simulink model "DriveSystemControl"  (R2023b)
settings: Solver=FixedStepAuto  StartTime=0.0  StopTime=Inf  FixedStep=0.001  RelTol=1e-3
PostLoadFcn:
  | if any(exist('dsrtsu_mdlpostloadfcn', 'file') ~= 0), dsrtsu_mdlpostloadfcn('Execute', bdroot); end
InitFcn:
  | , if any(exist('rtifpga_mdlclblib', 'file') ~= 0), rtifpga_mdlclblib('Init', bdroot); end,
  | , if any(exist('dsmpb_private', 'file') ~= 0), dsmpb_private('dsmpb_mdlclblib', 'Init', bdroot); end,
libraries: dsmpblib x2
(part 5 of 11)

== system DriveSystemControl/Bus Configuration (1) - Out/Manipulation/Virya Controller CAN File 08082024/WIP/CANChannel/PDUs/TCU03/sigSupervisorFault ==
  sigSupervisorFault : Inport
  Feature Switch : Subsystem
  _sigSupervisorFault_ : BusSelector  OutputSignals=Feature Switch
  wires:
  sigSupervisorFault/1 -> _sigSupervisorFault_/1  "sigSupervisorFault"
  _sigSupervisorFault_/1 -> Feature Switch/1(Feature Switch)  "<Feature Switch>"

== system DriveSystemControl/Bus Configuration (1) - Out/Manipulation/Virya Controller CAN File 08082024/WIP/CANChannel/PDUs/TCU03/sigThrottlewiperHigh ==
  sigThrottlewiperHigh : Inport
  Feature Switch : Subsystem
  _sigThrottlewiperHigh_ : BusSelector  OutputSignals=Feature Switch
  wires:
  sigThrottlewiperHigh/1 -> _sigThrottlewiperHigh_/1  "sigThrottlewiperHigh"
  _sigThrottlewiperHigh_/1 -> Feature Switch/1(Feature Switch)  "<Feature Switch>"

== system DriveSystemControl/Bus Configuration (1) - Out/Manipulation/Virya Controller CAN File 08082024/WIP/CANChannel/PDUs/TCU03/sigThrottlewiperLow ==
  sigThrottlewiperLow : Inport
  Feature Switch : Subsystem
  _sigThrottlewiperLow_ : BusSelector  OutputSignals=Feature Switch
  wires:
  sigThrottlewiperLow/1 -> _sigThrottlewiperLow_/1  "sigThrottlewiperLow"
  _sigThrottlewiperLow_/1 -> Feature Switch/1(Feature Switch)  "<Feature Switch>"

== system DriveSystemControl/Bus Configuration (1) - Out/Manipulation/Virya Controller CAN File 08082024/WIP/CANChannel/PDUs/TCU03/sigVCLRunTimeError ==
  sigVCLRunTimeError : Inport
  Feature Switch : Subsystem
  _sigVCLRunTimeError_ : BusSelector  OutputSignals=Feature Switch
  wires:
  sigVCLRunTimeError/1 -> _sigVCLRunTimeError_/1  "sigVCLRunTimeError"
  _sigVCLRunTimeError_/1 -> Feature Switch/1(Feature Switch)  "<Feature Switch>"

== system DriveSystemControl/Bus Configuration (1) - Out/Manipulation/Virya Controller CAN File 08082024/WIP/CANChannel/PDUs/TCU04/sigMCU5_DriveMode ==
  sigMCU5_DriveMode : Inport
  Feature Switch : Subsystem
  _sigMCU5_DriveMode_ : BusSelector  OutputSignals=Feature Switch
  wires:
  sigMCU5_DriveMode/1 -> _sigMCU5_DriveMode_/1  "sigMCU5_DriveMode"
  _sigMCU5_DriveMode_/1 -> Feature Switch/1(Feature Switch)  "<Feature Switch>"

== system DriveSystemControl/Bus Configuration (1) - Out/Manipulation/Virya Controller CAN File 08082024/WIP/CANChannel/PDUs/TCU04/sigMCU5_Efficiency ==
  sigMCU5_Efficiency : Inport
  Feature Switch : Subsystem
  _sigMCU5_Efficiency_ : BusSelector  OutputSignals=Feature Switch
  wires:
  sigMCU5_Efficiency/1 -> _sigMCU5_Efficiency_/1  "sigMCU5_Efficiency"
  _sigMCU5_Efficiency_/1 -> Feature Switch/1(Feature Switch)  "<Feature Switch>"

== system DriveSystemControl/Bus Configuration (1) - Out/Manipulation/Virya Controller CAN File 08082024/WIP/CANChannel/PDUs/TCU04/sigMCU5_Hillhold ==
  sigMCU5_Hillhold : Inport
  Feature Switch : Subsystem
  _sigMCU5_Hillhold_ : BusSelector  OutputSignals=Feature Switch
  wires:
  sigMCU5_Hillhold/1 -> _sigMCU5_Hillhold_/1  "sigMCU5_Hillhold"
  _sigMCU5_Hillhold_/1 -> Feature Switch/1(Feature Switch)  "<Feature Switch>"

== system DriveSystemControl/Bus Configuration (1) - Out/Manipulation/Virya Controller CAN File 08082024/WIP/CANChannel/PDUs/TCU04/sigMCU5_RegenFlag ==
  sigMCU5_RegenFlag : Inport
  Feature Switch : Subsystem
  _sigMCU5_RegenFlag_ : BusSelector  OutputSignals=Feature Switch
  wires:
  sigMCU5_RegenFlag/1 -> _sigMCU5_RegenFlag_/1  "sigMCU5_RegenFlag"
  _sigMCU5_RegenFlag_/1 -> Feature Switch/1(Feature Switch)  "<Feature Switch>"

== system DriveSystemControl/Bus Configuration (1) - Out/Manipulation/Virya Controller CAN File 08082024/WIP/CANChannel/PDUs/TCU04/sigMCU5_Speed ==
  sigMCU5_Speed : Inport
  Feature Switch : Subsystem
  _sigMCU5_Speed_ : BusSelector  OutputSignals=Feature Switch
  wires:
  sigMCU5_Speed/1 -> _sigMCU5_Speed_/1  "sigMCU5_Speed"
  _sigMCU5_Speed_/1 -> Feature Switch/1(Feature Switch)  "<Feature Switch>"

== system DriveSystemControl/Bus Configuration (1) - Out/Manipulation/Virya Controller CAN File 08082024/WIP/CANChannel/PDUs/TCU05/sigMCU6_Odometer ==
  sigMCU6_Odometer : Inport
  Feature Switch : Subsystem
  _sigMCU6_Odometer_ : BusSelector  OutputSignals=Feature Switch
  wires:
  sigMCU6_Odometer/1 -> _sigMCU6_Odometer_/1  "sigMCU6_Odometer"
  _sigMCU6_Odometer_/1 -> Feature Switch/1(Feature Switch)  "<Feature Switch>"

== system DriveSystemControl/Bus Configuration (1) - Out/Simulated ECUs/Virya Controller CAN File 08082024/BMS/RX/PDUs/TCU04/sigMCU5_DriveMode ==
  sigMCU5_DriveMode : Inport
  ISignal Value : Subsystem
  _sigMCU5_DriveMode_ : BusSelector  OutputSignals=ISignal Value
  wires:
  sigMCU5_DriveMode/1 -> _sigMCU5_DriveMode_/1  "sigMCU5_DriveMode"
  _sigMCU5_DriveMode_/1 -> ISignal Value/1(ISignal Value)  "<ISignal Value>"

== system DriveSystemControl/Bus Configuration (1) - Out/Simulated ECUs/Virya Controller CAN File 08082024/BMS/RX/PDUs/TCU04/sigMCU5_Efficiency ==
  sigMCU5_Efficiency : Inport
  ISignal Value : Subsystem
  _sigMCU5_Efficiency_ : BusSelector  OutputSignals=ISignal Value
  wires:
  sigMCU5_Efficiency/1 -> _sigMCU5_Efficiency_/1  "sigMCU5_Efficiency"
  _sigMCU5_Efficiency_/1 -> ISignal Value/1(ISignal Value)  "<ISignal Value>"

== system DriveSystemControl/Bus Configuration (1) - Out/Simulated ECUs/Virya Controller CAN File 08082024/BMS/RX/PDUs/TCU04/sigMCU5_Hillhold ==
  sigMCU5_Hillhold : Inport
  ISignal Value : Subsystem
  _sigMCU5_Hillhold_ : BusSelector  OutputSignals=ISignal Value
  wires:
  sigMCU5_Hillhold/1 -> _sigMCU5_Hillhold_/1  "sigMCU5_Hillhold"
  _sigMCU5_Hillhold_/1 -> ISignal Value/1(ISignal Value)  "<ISignal Value>"

== system DriveSystemControl/Bus Configuration (1) - Out/Simulated ECUs/Virya Controller CAN File 08082024/BMS/RX/PDUs/TCU04/sigMCU5_RegenFlag ==
  sigMCU5_RegenFlag : Inport
  ISignal Value : Subsystem
  _sigMCU5_RegenFlag_ : BusSelector  OutputSignals=ISignal Value
  wires:
  sigMCU5_RegenFlag/1 -> _sigMCU5_RegenFlag_/1  "sigMCU5_RegenFlag"
  _sigMCU5_RegenFlag_/1 -> ISignal Value/1(ISignal Value)  "<ISignal Value>"

== system DriveSystemControl/Bus Configuration (1) - Out/Simulated ECUs/Virya Controller CAN File 08082024/BMS/RX/PDUs/TCU04/sigMCU5_Speed ==
  sigMCU5_Speed : Inport
  ISignal Value : Subsystem
  _sigMCU5_Speed_ : BusSelector  OutputSignals=ISignal Value
  wires:
  sigMCU5_Speed/1 -> _sigMCU5_Speed_/1  "sigMCU5_Speed"
  _sigMCU5_Speed_/1 -> ISignal Value/1(ISignal Value)  "<ISignal Value>"

== system DriveSystemControl/Bus Configuration (1) - Out/Simulated ECUs/Virya Controller CAN File 08082024/IPC/RX/PDUs/BMS01/sigBatteryMalfunctionLight ==
  sigBatteryMalfunctionLight : Inport
  ISignal Value : Subsystem
  _sigBatteryMalfunctionLight_ : BusSelector  OutputSignals=ISignal Value
  wires:
  sigBatteryMalfunctionLight/1 -> _sigBatteryMalfunctionLight_/1  "sigBatteryMalfunctionLight"
  _sigBatteryMalfunctionLight_/1 -> ISignal Value/1(ISignal Value)  "<ISignal Value>"

== system DriveSystemControl/Bus Configuration (1) - Out/Simulated ECUs/Virya Controller CAN File 08082024/IPC/RX/PDUs/BMS01/sigKeyOnIndicator ==
  sigKeyOnIndicator : Inport
  ISignal Value : Subsystem
  _sigKeyOnIndicator_ : BusSelector  OutputSignals=ISignal Value
  wires:
  sigKeyOnIndicator/1 -> _sigKeyOnIndicator_/1  "sigKeyOnIndicator"
  _sigKeyOnIndicator_/1 -> ISignal Value/1(ISignal Value)  "<ISignal Value>"

== system DriveSystemControl/Bus Configuration (1) - Out/Simulated ECUs/Virya Controller CAN File 08082024/IPC/RX/PDUs/BMS01/sigStateOfCharge ==
  sigStateOfCharge : Inport
  ISignal Value : Subsystem
  _sigStateOfCharge_ : BusSelector  OutputSignals=ISignal Value
  wires:
  sigStateOfCharge/1 -> _sigStateOfCharge_/1  "sigStateOfCharge"
  _sigStateOfCharge_/1 -> ISignal Value/1(ISignal Value)  "<ISignal Value>"

== system DriveSystemControl/Bus Configuration (1) - Out/Simulated ECUs/Virya Controller CAN File 08082024/IPC/RX/PDUs/TCU01/sigBrake ==
  sigBrake : Inport
  ISignal Value : Subsystem
  _sigBrake_ : BusSelector  OutputSignals=ISignal Value
  wires:
  sigBrake/1 -> _sigBrake_/1  "sigBrake"
  _sigBrake_/1 -> ISignal Value/1(ISignal Value)  "<ISignal Value>"

== system DriveSystemControl/Bus Configuration (1) - Out/Simulated ECUs/Virya Controller CAN File 08082024/IPC/RX/PDUs/TCU01/sigControllerTemperature ==
  sigControllerTemperature : Inport
  ISignal Value : Subsystem
  _sigControllerTemperature_ : BusSelector  OutputSignals=ISignal Value
  wires:
  sigControllerTemperature/1 -> _sigControllerTemperature_/1  "sigControllerTemperature"
  _sigControllerTemperature_/1 -> ISignal Value/1(ISignal Value)  "<ISignal Value>"

== system DriveSystemControl/Bus Configuration (1) - Out/Simulated ECUs/Virya Controller CAN File 08082024/IPC/RX/PDUs/TCU01/sigDriveMode ==
  sigDriveMode : Inport
  ISignal Value : Subsystem
  _sigDriveMode_ : BusSelector  OutputSignals=ISignal Value
  wires:
  sigDriveMode/1 -> _sigDriveMode_/1  "sigDriveMode"
  _sigDriveMode_/1 -> ISignal Value/1(ISignal Value)  "<ISignal Value>"

== system DriveSystemControl/Bus Configuration (1) - Out/Simulated ECUs/Virya Controller CAN File 08082024/IPC/RX/PDUs/TCU01/sigMotorTemperature ==
  sigMotorTemperature : Inport
  ISignal Value : Subsystem
  _sigMotorTemperature_ : BusSelector  OutputSignals=ISignal Value
  wires:
  sigMotorTemperature/1 -> _sigMotorTemperature_/1  "sigMotorTemperature"
  _sigMotorTemperature_/1 -> ISignal Value/1(ISignal Value)  "<ISignal Value>"

== system DriveSystemControl/Bus Configuration (1) - Out/Simulated ECUs/Virya Controller CAN File 08082024/IPC/RX/PDUs/TCU01/sigRMSCurrent ==
  sigRMSCurrent : Inport
  ISignal Value : Subsystem
  _sigRMSCurrent_ : BusSelector  OutputSignals=ISignal Value
  wires:
  sigRMSCurrent/1 -> _sigRMSCurrent_/1  "sigRMSCurrent"
  _sigRMSCurrent_/1 -> ISignal Value/1(ISignal Value)  "<ISignal Value>"

== system DriveSystemControl/Bus Configuration (1) - Out/Simulated ECUs/Virya Controller CAN File 08082024/IPC/RX/PDUs/TCU01/sigSpeed ==
  sigSpeed : Inport
  ISignal Value : Subsystem
  _sigSpeed_ : BusSelector  OutputSignals=ISignal Value
  wires:
  sigSpeed/1 -> _sigSpeed_/1  "sigSpeed"
  _sigSpeed_/1 -> ISignal Value/1(ISignal Value)  "<ISignal Value>"

== system DriveSystemControl/Bus Configuration (1) - Out/Simulated ECUs/Virya Controller CAN File 08082024/IPC/RX/PDUs/TCU01/sigThrottle ==
  sigThrottle : Inport
  ISignal Value : Subsystem
  _sigThrottle_ : BusSelector  OutputSignals=ISignal Value
  wires:
  sigThrottle/1 -> _sigThrottle_/1  "sigThrottle"
  _sigThrottle_/1 -> ISignal Value/1(ISignal Value)  "<ISignal Value>"

== system DriveSystemControl/Bus Configuration (1) - Out/Simulated ECUs/Virya Controller CAN File 08082024/IPC/RX/PDUs/TCU03/Controller_CompleteFaults ==
  Controller_CompleteFaults : Inport
  ISignal Value : Subsystem
  _Controller_CompleteFaults_ : BusSelector  OutputSignals=ISignal Value
  wires:
  Controller_CompleteFaults/1 -> _Controller_CompleteFaults_/1  "Controller_CompleteFaults"
  _Controller_CompleteFaults_/1 -> ISignal Value/1(ISignal Value)  "<ISignal Value>"

== system DriveSystemControl/Bus Configuration (1) - Out/Simulated ECUs/Virya Controller CAN File 08082024/IPC/RX/PDUs/TCU03/sig5VSupplyFailure ==
  sig5VSupplyFailure : Inport
  ISignal Value : Subsystem
  _sig5VSupplyFailure_ : BusSelector  OutputSignals=ISignal Value
  wires:
  sig5VSupplyFailure/1 -> _sig5VSupplyFailure_/1  "sig5VSupplyFailure"
  _sig5VSupplyFailure_/1 -> ISignal Value/1(ISignal Value)  "<ISignal Value>"

== system DriveSystemControl/Bus Configuration (1) - Out/Simulated ECUs/Virya Controller CAN File 08082024/IPC/RX/PDUs/TCU03/sigBPosOvervoltageCutback ==
  sigBPosOvervoltageCutback : Inport
  ISignal Value : Subsystem
  _sigBPosOvervoltageCutback_ : BusSelector  OutputSignals=ISignal Value
  wires:
  sigBPosOvervoltageCutback/1 -> _sigBPosOvervoltageCutback_/1  "sigBPosOvervoltageCutback"
  _sigBPosOvervoltageCutback_/1 -> ISignal Value/1(ISignal Value)  "<ISignal Value>"

== system DriveSystemControl/Bus Configuration (1) - Out/Simulated ECUs/Virya Controller CAN File 08082024/IPC/RX/PDUs/TCU03/sigBPosUndervoltageCutback ==
  sigBPosUndervoltageCutback : Inport
  ISignal Value : Subsystem
  _sigBPosUndervoltageCutback_ : BusSelector  OutputSignals=ISignal Value
  wires:
  sigBPosUndervoltageCutback/1 -> _sigBPosUndervoltageCutback_/1  "sigBPosUndervoltageCutback"
  _sigBPosUndervoltageCutback_/1 -> ISignal Value/1(ISignal Value)  "<ISignal Value>"

== system DriveSystemControl/Bus Configuration (1) - Out/Simulated ECUs/Virya Controller CAN File 08082024/IPC/RX/PDUs/TCU03/sigBadCalibration ==
  sigBadCalibration : Inport
  ISignal Value : Subsystem
  _sigBadCalibration_ : BusSelector  OutputSignals=ISignal Value
  wires:
  sigBadCalibration/1 -> _sigBadCalibration_/1  "sigBadCalibration"
  _sigBadCalibration_/1 -> ISignal Value/1(ISignal Value)  "<ISignal Value>"

== system DriveSystemControl/Bus Configuration (1) - Out/Simulated ECUs/Virya Controller CAN File 08082024/IPC/RX/PDUs/TCU03/sigBrakeWiperHigh ==
  sigBrakeWiperHigh : Inport
  ISignal Value : Subsystem
  _sigBrakeWiperHigh_ : BusSelector  OutputSignals=ISignal Value
  wires:
  sigBrakeWiperHigh/1 -> _sigBrakeWiperHigh_/1  "sigBrakeWiperHigh"
  _sigBrakeWiperHigh_/1 -> ISignal Value/1(ISignal Value)  "<ISignal Value>"

== system DriveSystemControl/Bus Configuration (1) - Out/Simulated ECUs/Virya Controller CAN File 08082024/IPC/RX/PDUs/TCU03/sigBrakeWiperLow ==
  sigBrakeWiperLow : Inport
  ISignal Value : Subsystem
  _sigBrakeWiperLow_ : BusSelector  OutputSignals=ISignal Value
  wires:
  sigBrakeWiperLow/1 -> _sigBrakeWiperLow_/1  "sigBrakeWiperLow"
  _sigBrakeWiperLow_/1 -> ISignal Value/1(ISignal Value)  "<ISignal Value>"

== system DriveSystemControl/Bus Configuration (1) - Out/Simulated ECUs/Virya Controller CAN File 08082024/IPC/RX/PDUs/TCU03/sigCoil2DriverOpenShort ==
  sigCoil2DriverOpenShort : Inport
  ISignal Value : Subsystem
  _sigCoil2DriverOpenShort_ : BusSelector  OutputSignals=ISignal Value
  wires:
  sigCoil2DriverOpenShort/1 -> _sigCoil2DriverOpenShort_/1  "sigCoil2DriverOpenShort"
  _sigCoil2DriverOpenShort_/1 -> ISignal Value/1(ISignal Value)  "<ISignal Value>"

== system DriveSystemControl/Bus Configuration (1) - Out/Simulated ECUs/Virya Controller CAN File 08082024/IPC/RX/PDUs/TCU03/sigCoil3DriverOpenShort ==
  sigCoil3DriverOpenShort : Inport
  ISignal Value : Subsystem
  _sigCoil3DriverOpenShort_ : BusSelector  OutputSignals=ISignal Value
  wires:
  sigCoil3DriverOpenShort/1 -> _sigCoil3DriverOpenShort_/1  "sigCoil3DriverOpenShort"
  _sigCoil3DriverOpenShort_/1 -> ISignal Value/1(ISignal Value)  "<ISignal Value>"

== system DriveSystemControl/Bus Configuration (1) - Out/Simulated ECUs/Virya Controller CAN File 08082024/IPC/RX/PDUs/TCU03/sigCoil4DriverOpenShort ==
  sigCoil4DriverOpenShort : Inport
  ISignal Value : Subsystem
  _sigCoil4DriverOpenShort_ : BusSelector  OutputSignals=ISignal Value
  wires:
  sigCoil4DriverOpenShort/1 -> _sigCoil4DriverOpenShort_/1  "sigCoil4DriverOpenShort"
  _sigCoil4DriverOpenShort_/1 -> ISignal Value/1(ISignal Value)  "<ISignal Value>"

== system DriveSystemControl/Bus Configuration (1) - Out/Simulated ECUs/Virya Controller CAN File 08082024/IPC/RX/PDUs/TCU03/sigControllerCommonFault ==
  sigControllerCommonFault : Inport
  ISignal Value : Subsystem
  _sigControllerCommonFault_ : BusSelector  OutputSignals=ISignal Value
  wires:
  sigControllerCommonFault/1 -> _sigControllerCommonFault_/1  "sigControllerCommonFault"
  _sigControllerCommonFault_/1 -> ISignal Value/1(ISignal Value)  "<ISignal Value>"

== system DriveSystemControl/Bus Configuration (1) - Out/Simulated ECUs/Virya Controller CAN File 08082024/IPC/RX/PDUs/TCU03/sigControllerOverCurrent ==
  sigControllerOverCurrent : Inport
  ISignal Value : Subsystem
  _sigControllerOverCurrent_ : BusSelector  OutputSignals=ISignal Value
  wires:
  sigControllerOverCurrent/1 -> _sigControllerOverCurrent_/1  "sigControllerOverCurrent"
  _sigControllerOverCurrent_/1 -> ISignal Value/1(ISignal Value)  "<ISignal Value>"

== system DriveSystemControl/Bus Configuration (1) - Out/Simulated ECUs/Virya Controller CAN File 08082024/IPC/RX/PDUs/TCU03/sigControllerOvertempCutback ==
  sigControllerOvertempCutback : Inport
  ISignal Value : Subsystem
  _sigControllerOvertempCutback_ : BusSelector  OutputSignals=ISignal Value
  wires:
  sigControllerOvertempCutback/1 -> _sigControllerOvertempCutback_/1  "sigControllerOvertempCutback"
  _sigControllerOvertempCutback_/1 -> ISignal Value/1(ISignal Value)  "<ISignal Value>"

== system DriveSystemControl/Bus Configuration (1) - Out/Simulated ECUs/Virya Controller CAN File 08082024/IPC/RX/PDUs/TCU03/sigControllerSevereOvertemp ==
  sigControllerSevereOvertemp : Inport
  ISignal Value : Subsystem
  _sigControllerSevereOvertemp_ : BusSelector  OutputSignals=ISignal Value
  wires:
  sigControllerSevereOvertemp/1 -> _sigControllerSevereOvertemp_/1  "sigControllerSevereOvertemp"
  _sigControllerSevereOvertemp_/1 -> ISignal Value/1(ISignal Value)  "<ISignal Value>"

== system DriveSystemControl/Bus Configuration (1) - Out/Simulated ECUs/Virya Controller CAN File 08082024/IPC/RX/PDUs/TCU03/sigControllerSevereUndertemp ==
  sigControllerSevereUndertemp : Inport
  ISignal Value : Subsystem
  _sigControllerSevereUndertemp_ : BusSelector  OutputSignals=ISignal Value
  wires:
  sigControllerSevereUndertemp/1 -> _sigControllerSevereUndertemp_/1  "sigControllerSevereUndertemp"
  _sigControllerSevereUndertemp_/1 -> ISignal Value/1(ISignal Value)  "<ISignal Value>"

== system DriveSystemControl/Bus Configuration (1) - Out/Simulated ECUs/Virya Controller CAN File 08082024/IPC/RX/PDUs/TCU03/sigCurrentSensorFault ==
  sigCurrentSensorFault : Inport
  ISignal Value : Subsystem
  _sigCurrentSensorFault_ : BusSelector  OutputSignals=ISignal Value
  wires:
  sigCurrentSensorFault/1 -> _sigCurrentSensorFault_/1  "sigCurrentSensorFault"
  _sigCurrentSensorFault_/1 -> ISignal Value/1(ISignal Value)  "<ISignal Value>"

== system DriveSystemControl/Bus Configuration (1) - Out/Simulated ECUs/Virya Controller CAN File 08082024/IPC/RX/PDUs/TCU03/sigEEPROMFailure ==
  sigEEPROMFailure : Inport
  ISignal Value : Subsystem
  _sigEEPROMFailure_ : BusSelector  OutputSignals=ISignal Value
  wires:
  sigEEPROMFailure/1 -> _sigEEPROMFailure_/1  "sigEEPROMFailure"
  _sigEEPROMFailure_/1 -> ISignal Value/1(ISignal Value)  "<ISignal Value>"

== system DriveSystemControl/Bus Configuration (1) - Out/Simulated ECUs/Virya Controller CAN File 08082024/IPC/RX/PDUs/TCU03/sigHighPedalDisable ==
  sigHighPedalDisable : Inport
  ISignal Value : Subsystem
  _sigHighPedalDisable_ : BusSelector  OutputSignals=ISignal Value
  wires:
  sigHighPedalDisable/1 -> _sigHighPedalDisable_/1  "sigHighPedalDisable"
  _sigHighPedalDisable_/1 -> ISignal Value/1(ISignal Value)  "<ISignal Value>"

== system DriveSystemControl/Bus Configuration (1) - Out/Simulated ECUs/Virya Controller CAN File 08082024/IPC/RX/PDUs/TCU03/sigInsulationResistanceLow ==
  sigInsulationResistanceLow : Inport
  ISignal Value : Subsystem
  _sigInsulationResistanceLow_ : BusSelector  OutputSignals=ISignal Value
  wires:
  sigInsulationResistanceLow/1 -> _sigInsulationResistanceLow_/1  "sigInsulationResistanceLow"
  _sigInsulationResistanceLow_/1 -> ISignal Value/1(ISignal Value)  "<ISignal Value>"

== system DriveSystemControl/Bus Configuration (1) - Out/Simulated ECUs/Virya Controller CAN File 08082024/IPC/RX/PDUs/TCU03/sigMainContactorWelded ==
  sigMainContactorWelded : Inport
  ISignal Value : Subsystem
  _sigMainContactorWelded_ : BusSelector  OutputSignals=ISignal Value
  wires:
  sigMainContactorWelded/1 -> _sigMainContactorWelded_/1  "sigMainContactorWelded"
  _sigMainContactorWelded_/1 -> ISignal Value/1(ISignal Value)  "<ISignal Value>"

== system DriveSystemControl/Bus Configuration (1) - Out/Simulated ECUs/Virya Controller CAN File 08082024/IPC/RX/PDUs/TCU03/sigMainContactordidnotClose ==
  sigMainContactordidnotClose : Inport
  ISignal Value : Subsystem
  _sigMainContactordidnotClose_ : BusSelector  OutputSignals=ISignal Value
  wires:
  sigMainContactordidnotClose/1 -> _sigMainContactordidnotClose_/1  "sigMainContactordidnotClose"
  _sigMainContactordidnotClose_/1 -> ISignal Value/1(ISignal Value)  "<ISignal Value>"

== system DriveSystemControl/Bus Configuration (1) - Out/Simulated ECUs/Virya Controller CAN File 08082024/IPC/RX/PDUs/TCU03/sigMainOpenShort ==
  sigMainOpenShort : Inport
  ISignal Value : Subsystem
  _sigMainOpenShort_ : BusSelector  OutputSignals=ISignal Value
  wires:
  sigMainOpenShort/1 -> _sigMainOpenShort_/1  "sigMainOpenShort"
  _sigMainOpenShort_/1 -> ISignal Value/1(ISignal Value)  "<ISignal Value>"

== system DriveSystemControl/Bus Configuration (1) - Out/Simulated ECUs/Virya Controller CAN File 08082024/IPC/RX/PDUs/TCU03/sigMotorCharacterization ==
  sigMotorCharacterization : Inport
  ISignal Value : Subsystem
  _sigMotorCharacterization_ : BusSelector  OutputSignals=ISignal Value
  wires:
  sigMotorCharacterization/1 -> _sigMotorCharacterization_/1  "sigMotorCharacterization"
  _sigMotorCharacterization_/1 -> ISignal Value/1(ISignal Value)  "<ISignal Value>"

== system DriveSystemControl/Bus Configuration (1) - Out/Simulated ECUs/Virya Controller CAN File 08082024/IPC/RX/PDUs/TCU03/sigMotorPhaseOpen ==
  sigMotorPhaseOpen : Inport
  ISignal Value : Subsystem
  _sigMotorPhaseOpen_ : BusSelector  OutputSignals=ISignal Value
  wires:
  sigMotorPhaseOpen/1 -> _sigMotorPhaseOpen_/1  "sigMotorPhaseOpen"
  _sigMotorPhaseOpen_/1 -> ISignal Value/1(ISignal Value)  "<ISignal Value>"

== system DriveSystemControl/Bus Configuration (1) - Out/Simulated ECUs/Virya Controller CAN File 08082024/IPC/RX/PDUs/TCU03/sigMotorTempHotCutback ==
  sigMotorTempHotCutback : Inport
  ISignal Value : Subsystem
  _sigMotorTempHotCutback_ : BusSelector  OutputSignals=ISignal Value
  wires:
  sigMotorTempHotCutback/1 -> _sigMotorTempHotCutback_/1  "sigMotorTempHotCutback"
  _sigMotorTempHotCutback_/1 -> ISignal Value/1(ISignal Value)  "<ISignal Value>"

== system DriveSystemControl/Bus Configuration (1) - Out/Simulated ECUs/Virya Controller CAN File 08082024/IPC/RX/PDUs/TCU03/sigMotorTempSensorFault ==
  sigMotorTempSensorFault : Inport
  ISignal Value : Subsystem
  _sigMotorTempSensorFault_ : BusSelector  OutputSignals=ISignal Value
  wires:
  sigMotorTempSensorFault/1 -> _sigMotorTempSensorFault_/1  "sigMotorTempSensorFault"
  _sigMotorTempSensorFault_/1 -> ISignal Value/1(ISignal Value)  "<ISignal Value>"

== system DriveSystemControl/Bus Configuration (1) - Out/Simulated ECUs/Virya Controller CAN File 08082024/IPC/RX/PDUs/TCU03/sigOEM_BatterySTOPSignal ==
  sigOEM_BatterySTOPSignal : Inport
  ISignal Value : Subsystem
  _sigOEM_BatterySTOPSignal_ : BusSelector  OutputSignals=ISignal Value
  wires:
  sigOEM_BatterySTOPSignal/1 -> _sigOEM_BatterySTOPSignal_/1  "sigOEM_BatterySTOPSignal"
  _sigOEM_BatterySTOPSignal_/1 -> ISignal Value/1(ISignal Value)  "<ISignal Value>"

== system DriveSystemControl/Bus Configuration (1) - Out/Simulated ECUs/Virya Controller CAN File 08082024/IPC/RX/PDUs/TCU03/sigOEM_NoBatteryCAN ==
  sigOEM_NoBatteryCAN : Inport
  ISignal Value : Subsystem
  _sigOEM_NoBatteryCAN_ : BusSelector  OutputSignals=ISignal Value
  wires:
  sigOEM_NoBatteryCAN/1 -> _sigOEM_NoBatteryCAN_/1  "sigOEM_NoBatteryCAN"
  _sigOEM_NoBatteryCAN_/1 -> ISignal Value/1(ISignal Value)  "<ISignal Value>"

== system DriveSystemControl/Bus Configuration (1) - Out/Simulated ECUs/Virya Controller CAN File 08082024/IPC/RX/PDUs/TCU03/sigOSGeneral ==
  sigOSGeneral : Inport
  ISignal Value : Subsystem
  _sigOSGeneral_ : BusSelector  OutputSignals=ISignal Value
  wires:
  sigOSGeneral/1 -> _sigOSGeneral_/1  "sigOSGeneral"
  _sigOSGeneral_/1 -> ISignal Value/1(ISignal Value)  "<ISignal Value>"

== system DriveSystemControl/Bus Configuration (1) - Out/Simulated ECUs/Virya Controller CAN File 08082024/IPC/RX/PDUs/TCU03/sigPMACCommissioningNeeded ==
  sigPMACCommissioningNeeded : Inport
  ISignal Value : Subsystem
  _sigPMACCommissioningNeeded_ : BusSelector  OutputSignals=ISignal Value
  wires:
  sigPMACCommissioningNeeded/1 -> _sigPMACCommissioningNeeded_/1  "sigPMACCommissioningNeeded"
  _sigPMACCommissioningNeeded_/1 -> ISignal Value/1(ISignal Value)  "<ISignal Value>"

== system DriveSystemControl/Bus Configuration (1) - Out/Simulated ECUs/Virya Controller CAN File 08082024/IPC/RX/PDUs/TCU03/sigParameterChangeFault ==
  sigParameterChangeFault : Inport
  ISignal Value : Subsystem
  _sigParameterChangeFault_ : BusSelector  OutputSignals=ISignal Value
  wires:
  sigParameterChangeFault/1 -> _sigParameterChangeFault_/1  "sigParameterChangeFault"
  _sigParameterChangeFault_/1 -> ISignal Value/1(ISignal Value)  "<ISignal Value>"

== system DriveSystemControl/Bus Configuration (1) - Out/Simulated ECUs/Virya Controller CAN File 08082024/IPC/RX/PDUs/TCU03/sigPhasePWMMismatch ==
  sigPhasePWMMismatch : Inport
  ISignal Value : Subsystem
  _sigPhasePWMMismatch_ : BusSelector  OutputSignals=ISignal Value
  wires:
  sigPhasePWMMismatch/1 -> _sigPhasePWMMismatch_/1  "sigPhasePWMMismatch"
  _sigPhasePWMMismatch_/1 -> ISignal Value/1(ISignal Value)  "<ISignal Value>"

== system DriveSystemControl/Bus Configuration (1) - Out/Simulated ECUs/Virya Controller CAN File 08082024/IPC/RX/PDUs/TCU03/sigPrechargeFailed ==
  sigPrechargeFailed : Inport
  ISignal Value : Subsystem
  _sigPrechargeFailed_ : BusSelector  OutputSignals=ISignal Value
  wires:
  sigPrechargeFailed/1 -> _sigPrechargeFailed_/1  "sigPrechargeFailed"
  _sigPrechargeFailed_/1 -> ISignal Value/1(ISignal Value)  "<ISignal Value>"

== system DriveSystemControl/Bus Configuration (1) - Out/Simulated ECUs/Virya Controller CAN File 08082024/IPC/RX/PDUs/TCU03/sigSevereBPosOvervoltage ==
  sigSevereBPosOvervoltage : Inport
  ISignal Value : Subsystem
  _sigSevereBPosOvervoltage_ : BusSelector  OutputSignals=ISignal Value
  wires:
  sigSevereBPosOvervoltage/1 -> _sigSevereBPosOvervoltage_/1  "sigSevereBPosOvervoltage"
  _sigSevereBPosOvervoltage_/1 -> ISignal Value/1(ISignal Value)  "<ISignal Value>"

== system DriveSystemControl/Bus Configuration (1) - Out/Simulated ECUs/Virya Controller CAN File 08082024/IPC/RX/PDUs/TCU03/sigSevereBPosUndervoltage ==
  sigSevereBPosUndervoltage : Inport
  ISignal Value : Subsystem
  _sigSevereBPosUndervoltage_ : BusSelector  OutputSignals=ISignal Value
  wires:
  sigSevereBPosUndervoltage/1 -> _sigSevereBPosUndervoltage_/1  "sigSevereBPosUndervoltage"
  _sigSevereBPosUndervoltage_/1 -> ISignal Value/1(ISignal Value)  "<ISignal Value>"

== system DriveSystemControl/Bus Configuration (1) - Out/Simulated ECUs/Virya Controller CAN File 08082024/IPC/RX/PDUs/TCU03/sigSevereKSIOvervoltage ==
  sigSevereKSIOvervoltage : Inport
  ISignal Value : Subsystem
  _sigSevereKSIOvervoltage_ : BusSelector  OutputSignals=ISignal Value
  wires:
  sigSevereKSIOvervoltage/1 -> _sigSevereKSIOvervoltage_/1  "sigSevereKSIOvervoltage"
  _sigSevereKSIOvervoltage_/1 -> ISignal Value/1(ISignal Value)  "<ISignal Value>"

== system DriveSystemControl/Bus Configuration (1) - Out/Simulated ECUs/Virya Controller CAN File 08082024/IPC/RX/PDUs/TCU03/sigSevereKSIUndervoltage ==
  sigSevereKSIUndervoltage : Inport
  ISignal Value : Subsystem
  _sigSevereKSIUndervoltage_ : BusSelector  OutputSignals=ISignal Value
  wires:
  sigSevereKSIUndervoltage/1 -> _sigSevereKSIUndervoltage_/1  "sigSevereKSIUndervoltage"
  _sigSevereKSIUndervoltage_/1 -> ISignal Value/1(ISignal Value)  "<ISignal Value>"

== system DriveSystemControl/Bus Configuration (1) - Out/Simulated ECUs/Virya Controller CAN File 08082024/IPC/RX/PDUs/TCU03/sigSinCosMisalignment ==
  sigSinCosMisalignment : Inport
  ISignal Value : Subsystem
  _sigSinCosMisalignment_ : BusSelector  OutputSignals=ISignal Value
  wires:
  sigSinCosMisalignment/1 -> _sigSinCosMisalignment_/1  "sigSinCosMisalignment"
  _sigSinCosMisalignment_/1 -> ISignal Value/1(ISignal Value)  "<ISignal Value>"

== system DriveSystemControl/Bus Configuration (1) - Out/Simulated ECUs/Virya Controller CAN File 08082024/IPC/RX/PDUs/TCU03/sigSinCosSensorFault ==
  sigSinCosSensorFault : Inport
  ISignal Value : Subsystem
  _sigSinCosSensorFault_ : BusSelector  OutputSignals=ISignal Value
  wires:
  sigSinCosSensorFault/1 -> _sigSinCosSensorFault_/1  "sigSinCosSensorFault"
  _sigSinCosSensorFault_/1 -> ISignal Value/1(ISignal Value)  "<ISignal Value>"

== system DriveSystemControl/Bus Configuration (1) - Out/Simulated ECUs/Virya Controller CAN File 08082024/IPC/RX/PDUs/TCU03/sigStallDetected ==
  sigStallDetected : Inport
  ISignal Value : Subsystem
  _sigStallDetected_ : BusSelector  OutputSignals=ISignal Value
  wires:
  sigStallDetected/1 -> _sigStallDetected_/1  "sigStallDetected"
  _sigStallDetected_/1 -> ISignal Value/1(ISignal Value)  "<ISignal Value>"

== system DriveSystemControl/Bus Configuration (1) - Out/Simulated ECUs/Virya Controller CAN File 08082024/IPC/RX/PDUs/TCU03/sigSupervisorFault ==
  sigSupervisorFault : Inport
  ISignal Value : Subsystem
  _sigSupervisorFault_ : BusSelector  OutputSignals=ISignal Value
  wires:
  sigSupervisorFault/1 -> _sigSupervisorFault_/1  "sigSupervisorFault"
  _sigSupervisorFault_/1 -> ISignal Value/1(ISignal Value)  "<ISignal Value>"

== system DriveSystemControl/Bus Configuration (1) - Out/Simulated ECUs/Virya Controller CAN File 08082024/IPC/RX/PDUs/TCU03/sigThrottlewiperHigh ==
  sigThrottlewiperHigh : Inport
  ISignal Value : Subsystem
  _sigThrottlewiperHigh_ : BusSelector  OutputSignals=ISignal Value
  wires:
  sigThrottlewiperHigh/1 -> _sigThrottlewiperHigh_/1  "sigThrottlewiperHigh"
  _sigThrottlewiperHigh_/1 -> ISignal Value/1(ISignal Value)  "<ISignal Value>"

== system DriveSystemControl/Bus Configuration (1) - Out/Simulated ECUs/Virya Controller CAN File 08082024/IPC/RX/PDUs/TCU03/sigThrottlewiperLow ==
  sigThrottlewiperLow : Inport
  ISignal Value : Subsystem
  _sigThrottlewiperLow_ : BusSelector  OutputSignals=ISignal Value
  wires:
  sigThrottlewiperLow/1 -> _sigThrottlewiperLow_/1  "sigThrottlewiperLow"
  _sigThrottlewiperLow_/1 -> ISignal Value/1(ISignal Value)  "<ISignal Value>"

== system DriveSystemControl/Bus Configuration (1) - Out/Simulated ECUs/Virya Controller CAN File 08082024/IPC/RX/PDUs/TCU03/sigVCLRunTimeError ==
  sigVCLRunTimeError : Inport
  ISignal Value : Subsystem
  _sigVCLRunTimeError_ : BusSelector  OutputSignals=ISignal Value
  wires:
  sigVCLRunTimeError/1 -> _sigVCLRunTimeError_/1  "sigVCLRunTimeError"
  _sigVCLRunTimeError_/1 -> ISignal Value/1(ISignal Value)  "<ISignal Value>"

== system DriveSystemControl/Bus Configuration (1) - Out/Simulated ECUs/Virya Controller CAN File 08082024/IPC/RX/PDUs/TCU04/sigMCU5_DriveMode ==
  sigMCU5_DriveMode : Inport
  ISignal Value : Subsystem
  _sigMCU5_DriveMode_ : BusSelector  OutputSignals=ISignal Value
  wires:
  sigMCU5_DriveMode/1 -> _sigMCU5_DriveMode_/1  "sigMCU5_DriveMode"
  _sigMCU5_DriveMode_/1 -> ISignal Value/1(ISignal Value)  "<ISignal Value>"

== system DriveSystemControl/Bus Configuration (1) - Out/Simulated ECUs/Virya Controller CAN File 08082024/IPC/RX/PDUs/TCU04/sigMCU5_Efficiency ==
  sigMCU5_Efficiency : Inport
  ISignal Value : Subsystem
  _sigMCU5_Efficiency_ : BusSelector  OutputSignals=ISignal Value
  wires:
  sigMCU5_Efficiency/1 -> _sigMCU5_Efficiency_/1  "sigMCU5_Efficiency"
  _sigMCU5_Efficiency_/1 -> ISignal Value/1(ISignal Value)  "<ISignal Value>"

== system DriveSystemControl/Bus Configuration (1) - Out/Simulated ECUs/Virya Controller CAN File 08082024/IPC/RX/PDUs/TCU04/sigMCU5_Hillhold ==
  sigMCU5_Hillhold : Inport
  ISignal Value : Subsystem
  _sigMCU5_Hillhold_ : BusSelector  OutputSignals=ISignal Value
  wires:
  sigMCU5_Hillhold/1 -> _sigMCU5_Hillhold_/1  "sigMCU5_Hillhold"
  _sigMCU5_Hillhold_/1 -> ISignal Value/1(ISignal Value)  "<ISignal Value>"

== system DriveSystemControl/Bus Configuration (1) - Out/Simulated ECUs/Virya Controller CAN File 08082024/IPC/RX/PDUs/TCU04/sigMCU5_RegenFlag ==
  sigMCU5_RegenFlag : Inport
  ISignal Value : Subsystem
  _sigMCU5_RegenFlag_ : BusSelector  OutputSignals=ISignal Value
  wires:
  sigMCU5_RegenFlag/1 -> _sigMCU5_RegenFlag_/1  "sigMCU5_RegenFlag"
  _sigMCU5_RegenFlag_/1 -> ISignal Value/1(ISignal Value)  "<ISignal Value>"

== system DriveSystemControl/Bus Configuration (1) - Out/Simulated ECUs/Virya Controller CAN File 08082024/IPC/RX/PDUs/TCU04/sigMCU5_Speed ==
  sigMCU5_Speed : Inport
  ISignal Value : Subsystem
  _sigMCU5_Speed_ : BusSelector  OutputSignals=ISignal Value
  wires:
  sigMCU5_Speed/1 -> _sigMCU5_Speed_/1  "sigMCU5_Speed"
  _sigMCU5_Speed_/1 -> ISignal Value/1(ISignal Value)  "<ISignal Value>"

== system DriveSystemControl/Bus Configuration (1) - Out/Simulated ECUs/Virya Controller CAN File 08082024/IPC/RX/PDUs/TCU05/sigMCU6_Odometer ==
  sigMCU6_Odometer : Inport
  ISignal Value : Subsystem
  _sigMCU6_Odometer_ : BusSelector  OutputSignals=ISignal Value
  wires:
  sigMCU6_Odometer/1 -> _sigMCU6_Odometer_/1  "sigMCU6_Odometer"
  _sigMCU6_Odometer_/1 -> ISignal Value/1(ISignal Value)  "<ISignal Value>"

== system DriveSystemControl/Bus Configuration (1) - Out/Simulated ECUs/Virya Controller CAN File 08082024/TCU/RX/PDUs/BMS02/sigBatteryCurrent ==
  sigBatteryCurrent : Inport
  ISignal Value : Subsystem
  _sigBatteryCurrent_ : BusSelector  OutputSignals=ISignal Value
  wires:
  sigBatteryCurrent/1 -> _sigBatteryCurrent_/1  "sigBatteryCurrent"
  _sigBatteryCurrent_/1 -> ISignal Value/1(ISignal Value)  "<ISignal Value>"

== system DriveSystemControl/Bus Configuration (1) - Out/Simulated ECUs/Virya Controller CAN File 08082024/TCU/RX/PDUs/BMS02/sigDriveCurrentLimit ==
  sigDriveCurrentLimit : Inport
  ISignal Value : Subsystem
  _sigDriveCurrentLimit_ : BusSelector  OutputSignals=ISignal Value
  wires:
  sigDriveCurrentLimit/1 -> _sigDriveCurrentLimit_/1  "sigDriveCurrentLimit"
  _sigDriveCurrentLimit_/1 -> ISignal Value/1(ISignal Value)  "<ISignal Value>"

== system DriveSystemControl/Bus Configuration (1) - Out/Simulated ECUs/Virya Controller CAN File 08082024/TCU/RX/PDUs/BMS02/sigRegenCurrentLimit ==
  sigRegenCurrentLimit : Inport
  ISignal Value : Subsystem
  _sigRegenCurrentLimit_ : BusSelector  OutputSignals=ISignal Value
  wires:
  sigRegenCurrentLimit/1 -> _sigRegenCurrentLimit_/1  "sigRegenCurrentLimit"
  _sigRegenCurrentLimit_/1 -> ISignal Value/1(ISignal Value)  "<ISignal Value>"

== system DriveSystemControl/Bus Configuration (1) - Out/Simulated ECUs/Virya Controller CAN File 08082024/TCU/RX/PDUs/BMS02/sigVehicleModeRequest ==
  sigVehicleModeRequest : Inport
  ISignal Value : Subsystem
  _sigVehicleModeRequest_ : BusSelector  OutputSignals=ISignal Value
  wires:
  sigVehicleModeRequest/1 -> _sigVehicleModeRequest_/1  "sigVehicleModeRequest"
  _sigVehicleModeRequest_/1 -> ISignal Value/1(ISignal Value)  "<ISignal Value>"

== system DriveSystemControl/Bus Configuration (1) - Out/Simulated ECUs/Virya Controller CAN File 08082024/Telematics/RX/PDUs/BMS01/sigBatteryMalfunctionLight ==
  sigBatteryMalfunctionLight : Inport
  ISignal Value : Subsystem
  _sigBatteryMalfunctionLight_ : BusSelector  OutputSignals=ISignal Value
  wires:
  sigBatteryMalfunctionLight/1 -> _sigBatteryMalfunctionLight_/1  "sigBatteryMalfunctionLight"
  _sigBatteryMalfunctionLight_/1 -> ISignal Value/1(ISignal Value)  "<ISignal Value>"

== system DriveSystemControl/Bus Configuration (1) - Out/Simulated ECUs/Virya Controller CAN File 08082024/Telematics/RX/PDUs/BMS01/sigKeyOnIndicator ==
  sigKeyOnIndicator : Inport
  ISignal Value : Subsystem
  _sigKeyOnIndicator_ : BusSelector  OutputSignals=ISignal Value
  wires:
  sigKeyOnIndicator/1 -> _sigKeyOnIndicator_/1  "sigKeyOnIndicator"
  _sigKeyOnIndicator_/1 -> ISignal Value/1(ISignal Value)  "<ISignal Value>"

== system DriveSystemControl/Bus Configuration (1) - Out/Simulated ECUs/Virya Controller CAN File 08082024/Telematics/RX/PDUs/BMS01/sigStateOfCharge ==
  sigStateOfCharge : Inport
  ISignal Value : Subsystem
  _sigStateOfCharge_ : BusSelector  OutputSignals=ISignal Value
  wires:
  sigStateOfCharge/1 -> _sigStateOfCharge_/1  "sigStateOfCharge"
  _sigStateOfCharge_/1 -> ISignal Value/1(ISignal Value)  "<ISignal Value>"

== system DriveSystemControl/Bus Configuration (1) - Out/Simulated ECUs/Virya Controller CAN File 08082024/Telematics/RX/PDUs/BMS02/sigBatteryCurrent ==
  sigBatteryCurrent : Inport
  ISignal Value : Subsystem
  _sigBatteryCurrent_ : BusSelector  OutputSignals=ISignal Value
  wires:
  sigBatteryCurrent/1 -> _sigBatteryCurrent_/1  "sigBatteryCurrent"
  _sigBatteryCurrent_/1 -> ISignal Value/1(ISignal Value)  "<ISignal Value>"

== system DriveSystemControl/Bus Configuration (1) - Out/Simulated ECUs/Virya Controller CAN File 08082024/Telematics/RX/PDUs/BMS02/sigDriveCurrentLimit ==
  sigDriveCurrentLimit : Inport
  ISignal Value : Subsystem
  _sigDriveCurrentLimit_ : BusSelector  OutputSignals=ISignal Value
  wires:
  sigDriveCurrentLimit/1 -> _sigDriveCurrentLimit_/1  "sigDriveCurrentLimit"
  _sigDriveCurrentLimit_/1 -> ISignal Value/1(ISignal Value)  "<ISignal Value>"

== system DriveSystemControl/Bus Configuration (1) - Out/Simulated ECUs/Virya Controller CAN File 08082024/Telematics/RX/PDUs/BMS02/sigRegenCurrentLimit ==
  sigRegenCurrentLimit : Inport
  ISignal Value : Subsystem
  _sigRegenCurrentLimit_ : BusSelector  OutputSignals=ISignal Value
  wires:
  sigRegenCurrentLimit/1 -> _sigRegenCurrentLimit_/1  "sigRegenCurrentLimit"
  _sigRegenCurrentLimit_/1 -> ISignal Value/1(ISignal Value)  "<ISignal Value>"

== system DriveSystemControl/Bus Configuration (1) - Out/Simulated ECUs/Virya Controller CAN File 08082024/Telematics/RX/PDUs/BMS02/sigVehicleModeRequest ==
  sigVehicleModeRequest : Inport
  ISignal Value : Subsystem
  _sigVehicleModeRequest_ : BusSelector  OutputSignals=ISignal Value
  wires:
  sigVehicleModeRequest/1 -> _sigVehicleModeRequest_/1  "sigVehicleModeRequest"
  _sigVehicleModeRequest_/1 -> ISignal Value/1(ISignal Value)  "<ISignal Value>"

== system DriveSystemControl/Bus Configuration (1) - Out/Simulated ECUs/Virya Controller CAN File 08082024/Telematics/RX/PDUs/TCU01/sigBrake ==
  sigBrake : Inport
  ISignal Value : Subsystem
  _sigBrake_ : BusSelector  OutputSignals=ISignal Value
  wires:
  sigBrake/1 -> _sigBrake_/1  "sigBrake"
  _sigBrake_/1 -> ISignal Value/1(ISignal Value)  "<ISignal Value>"

== system DriveSystemControl/Bus Configuration (1) - Out/Simulated ECUs/Virya Controller CAN File 08082024/Telematics/RX/PDUs/TCU01/sigControllerTemperature ==
  sigControllerTemperature : Inport
  ISignal Value : Subsystem
  _sigControllerTemperature_ : BusSelector  OutputSignals=ISignal Value
  wires:
  sigControllerTemperature/1 -> _sigControllerTemperature_/1  "sigControllerTemperature"
  _sigControllerTemperature_/1 -> ISignal Value/1(ISignal Value)  "<ISignal Value>"

== system DriveSystemControl/Bus Configuration (1) - Out/Simulated ECUs/Virya Controller CAN File 08082024/Telematics/RX/PDUs/TCU01/sigDriveMode ==
  sigDriveMode : Inport
  ISignal Value : Subsystem
  _sigDriveMode_ : BusSelector  OutputSignals=ISignal Value
  wires:
  sigDriveMode/1 -> _sigDriveMode_/1  "sigDriveMode"
  _sigDriveMode_/1 -> ISignal Value/1(ISignal Value)  "<ISignal Value>"

== system DriveSystemControl/Bus Configuration (1) - Out/Simulated ECUs/Virya Controller CAN File 08082024/Telematics/RX/PDUs/TCU01/sigMotorTemperature ==
  sigMotorTemperature : Inport
  ISignal Value : Subsystem
  _sigMotorTemperature_ : BusSelector  OutputSignals=ISignal Value
  wires:
  sigMotorTemperature/1 -> _sigMotorTemperature_/1  "sigMotorTemperature"
  _sigMotorTemperature_/1 -> ISignal Value/1(ISignal Value)  "<ISignal Value>"

== system DriveSystemControl/Bus Configuration (1) - Out/Simulated ECUs/Virya Controller CAN File 08082024/Telematics/RX/PDUs/TCU01/sigRMSCurrent ==
  sigRMSCurrent : Inport
  ISignal Value : Subsystem
  _sigRMSCurrent_ : BusSelector  OutputSignals=ISignal Value
  wires:
  sigRMSCurrent/1 -> _sigRMSCurrent_/1  "sigRMSCurrent"
  _sigRMSCurrent_/1 -> ISignal Value/1(ISignal Value)  "<ISignal Value>"

== system DriveSystemControl/Bus Configuration (1) - Out/Simulated ECUs/Virya Controller CAN File 08082024/Telematics/RX/PDUs/TCU01/sigSpeed ==
  sigSpeed : Inport
  ISignal Value : Subsystem
  _sigSpeed_ : BusSelector  OutputSignals=ISignal Value
  wires:
  sigSpeed/1 -> _sigSpeed_/1  "sigSpeed"
  _sigSpeed_/1 -> ISignal Value/1(ISignal Value)  "<ISignal Value>"

== system DriveSystemControl/Bus Configuration (1) - Out/Simulated ECUs/Virya Controller CAN File 08082024/Telematics/RX/PDUs/TCU01/sigThrottle ==
  sigThrottle : Inport
  ISignal Value : Subsystem
  _sigThrottle_ : BusSelector  OutputSignals=ISignal Value
  wires:
  sigThrottle/1 -> _sigThrottle_/1  "sigThrottle"
  _sigThrottle_/1 -> ISignal Value/1(ISignal Value)  "<ISignal Value>"

== system DriveSystemControl/Bus Configuration (1) - Out/Simulated ECUs/Virya Controller CAN File 08082024/Telematics/RX/PDUs/TCU02/sigCapacitorVoltage ==
  sigCapacitorVoltage : Inport
  ISignal Value : Subsystem
  _sigCapacitorVoltage_ : BusSelector  OutputSignals=ISignal Value
  wires:
  sigCapacitorVoltage/1 -> _sigCapacitorVoltage_/1  "sigCapacitorVoltage"
  _sigCapacitorVoltage_/1 -> ISignal Value/1(ISignal Value)  "<ISignal Value>"

== system DriveSystemControl/Bus Configuration (1) - Out/Simulated ECUs/Virya Controller CAN File 08082024/Telematics/RX/PDUs/TCU02/sigMotorRPM ==
  sigMotorRPM : Inport
  ISignal Value : Subsystem
  _sigMotorRPM_ : BusSelector  OutputSignals=ISignal Value
  wires:
  sigMotorRPM/1 -> _sigMotorRPM_/1  "sigMotorRPM"
  _sigMotorRPM_/1 -> ISignal Value/1(ISignal Value)  "<ISignal Value>"

== system DriveSystemControl/Bus Configuration (1) - Out/Simulated ECUs/Virya Controller CAN File 08082024/Telematics/RX/PDUs/TCU02/sigOdometer ==
  sigOdometer : Inport
  ISignal Value : Subsystem
  _sigOdometer_ : BusSelector  OutputSignals=ISignal Value
  wires:
  sigOdometer/1 -> _sigOdometer_/1  "sigOdometer"
  _sigOdometer_/1 -> ISignal Value/1(ISignal Value)  "<ISignal Value>"

== system DriveSystemControl/Bus Configuration (1) - Out/Simulated ECUs/Virya Controller CAN File 08082024/Telematics/RX/PDUs/TCU03/Controller_CompleteFaults ==
  Controller_CompleteFaults : Inport
  ISignal Value : Subsystem
  _Controller_CompleteFaults_ : BusSelector  OutputSignals=ISignal Value
  wires:
  Controller_CompleteFaults/1 -> _Controller_CompleteFaults_/1  "Controller_CompleteFaults"
  _Controller_CompleteFaults_/1 -> ISignal Value/1(ISignal Value)  "<ISignal Value>"

== system DriveSystemControl/Bus Configuration (1) - Out/Simulated ECUs/Virya Controller CAN File 08082024/Telematics/RX/PDUs/TCU03/sig5VSupplyFailure ==
  sig5VSupplyFailure : Inport
  ISignal Value : Subsystem
  _sig5VSupplyFailure_ : BusSelector  OutputSignals=ISignal Value
  wires:
  sig5VSupplyFailure/1 -> _sig5VSupplyFailure_/1  "sig5VSupplyFailure"
  _sig5VSupplyFailure_/1 -> ISignal Value/1(ISignal Value)  "<ISignal Value>"

== system DriveSystemControl/Bus Configuration (1) - Out/Simulated ECUs/Virya Controller CAN File 08082024/Telematics/RX/PDUs/TCU03/sigBPosOvervoltageCutback ==
  sigBPosOvervoltageCutback : Inport
  ISignal Value : Subsystem
  _sigBPosOvervoltageCutback_ : BusSelector  OutputSignals=ISignal Value
  wires:
  sigBPosOvervoltageCutback/1 -> _sigBPosOvervoltageCutback_/1  "sigBPosOvervoltageCutback"
  _sigBPosOvervoltageCutback_/1 -> ISignal Value/1(ISignal Value)  "<ISignal Value>"

== system DriveSystemControl/Bus Configuration (1) - Out/Simulated ECUs/Virya Controller CAN File 08082024/Telematics/RX/PDUs/TCU03/sigBPosUndervoltageCutback ==
  sigBPosUndervoltageCutback : Inport
  ISignal Value : Subsystem
  _sigBPosUndervoltageCutback_ : BusSelector  OutputSignals=ISignal Value
  wires:
  sigBPosUndervoltageCutback/1 -> _sigBPosUndervoltageCutback_/1  "sigBPosUndervoltageCutback"
  _sigBPosUndervoltageCutback_/1 -> ISignal Value/1(ISignal Value)  "<ISignal Value>"

== system DriveSystemControl/Bus Configuration (1) - Out/Simulated ECUs/Virya Controller CAN File 08082024/Telematics/RX/PDUs/TCU03/sigBadCalibration ==
  sigBadCalibration : Inport
  ISignal Value : Subsystem
  _sigBadCalibration_ : BusSelector  OutputSignals=ISignal Value
  wires:
  sigBadCalibration/1 -> _sigBadCalibration_/1  "sigBadCalibration"
  _sigBadCalibration_/1 -> ISignal Value/1(ISignal Value)  "<ISignal Value>"

== system DriveSystemControl/Bus Configuration (1) - Out/Simulated ECUs/Virya Controller CAN File 08082024/Telematics/RX/PDUs/TCU03/sigBrakeWiperHigh ==
  sigBrakeWiperHigh : Inport
  ISignal Value : Subsystem
  _sigBrakeWiperHigh_ : BusSelector  OutputSignals=ISignal Value
  wires:
  sigBrakeWiperHigh/1 -> _sigBrakeWiperHigh_/1  "sigBrakeWiperHigh"
  _sigBrakeWiperHigh_/1 -> ISignal Value/1(ISignal Value)  "<ISignal Value>"

== system DriveSystemControl/Bus Configuration (1) - Out/Simulated ECUs/Virya Controller CAN File 08082024/Telematics/RX/PDUs/TCU03/sigBrakeWiperLow ==
  sigBrakeWiperLow : Inport
  ISignal Value : Subsystem
  _sigBrakeWiperLow_ : BusSelector  OutputSignals=ISignal Value
  wires:
  sigBrakeWiperLow/1 -> _sigBrakeWiperLow_/1  "sigBrakeWiperLow"
  _sigBrakeWiperLow_/1 -> ISignal Value/1(ISignal Value)  "<ISignal Value>"

== system DriveSystemControl/Bus Configuration (1) - Out/Simulated ECUs/Virya Controller CAN File 08082024/Telematics/RX/PDUs/TCU03/sigCoil2DriverOpenShort ==
  sigCoil2DriverOpenShort : Inport
  ISignal Value : Subsystem
  _sigCoil2DriverOpenShort_ : BusSelector  OutputSignals=ISignal Value
  wires:
  sigCoil2DriverOpenShort/1 -> _sigCoil2DriverOpenShort_/1  "sigCoil2DriverOpenShort"
  _sigCoil2DriverOpenShort_/1 -> ISignal Value/1(ISignal Value)  "<ISignal Value>"

== system DriveSystemControl/Bus Configuration (1) - Out/Simulated ECUs/Virya Controller CAN File 08082024/Telematics/RX/PDUs/TCU03/sigCoil3DriverOpenShort ==
  sigCoil3DriverOpenShort : Inport
  ISignal Value : Subsystem
  _sigCoil3DriverOpenShort_ : BusSelector  OutputSignals=ISignal Value
  wires:
  sigCoil3DriverOpenShort/1 -> _sigCoil3DriverOpenShort_/1  "sigCoil3DriverOpenShort"
  _sigCoil3DriverOpenShort_/1 -> ISignal Value/1(ISignal Value)  "<ISignal Value>"

== system DriveSystemControl/Bus Configuration (1) - Out/Simulated ECUs/Virya Controller CAN File 08082024/Telematics/RX/PDUs/TCU03/sigCoil4DriverOpenShort ==
  sigCoil4DriverOpenShort : Inport
  ISignal Value : Subsystem
  _sigCoil4DriverOpenShort_ : BusSelector  OutputSignals=ISignal Value
  wires:
  sigCoil4DriverOpenShort/1 -> _sigCoil4DriverOpenShort_/1  "sigCoil4DriverOpenShort"
  _sigCoil4DriverOpenShort_/1 -> ISignal Value/1(ISignal Value)  "<ISignal Value>"

== system DriveSystemControl/Bus Configuration (1) - Out/Simulated ECUs/Virya Controller CAN File 08082024/Telematics/RX/PDUs/TCU03/sigControllerCommonFault ==
  sigControllerCommonFault : Inport
  ISignal Value : Subsystem
  _sigControllerCommonFault_ : BusSelector  OutputSignals=ISignal Value
  wires:
  sigControllerCommonFault/1 -> _sigControllerCommonFault_/1  "sigControllerCommonFault"
  _sigControllerCommonFault_/1 -> ISignal Value/1(ISignal Value)  "<ISignal Value>"

== system DriveSystemControl/Bus Configuration (1) - Out/Simulated ECUs/Virya Controller CAN File 08082024/Telematics/RX/PDUs/TCU03/sigControllerOverCurrent ==
  sigControllerOverCurrent : Inport
  ISignal Value : Subsystem
  _sigControllerOverCurrent_ : BusSelector  OutputSignals=ISignal Value
  wires:
  sigControllerOverCurrent/1 -> _sigControllerOverCurrent_/1  "sigControllerOverCurrent"
  _sigControllerOverCurrent_/1 -> ISignal Value/1(ISignal Value)  "<ISignal Value>"

== system DriveSystemControl/Bus Configuration (1) - Out/Simulated ECUs/Virya Controller CAN File 08082024/Telematics/RX/PDUs/TCU03/sigControllerOvertempCutback ==
  sigControllerOvertempCutback : Inport
  ISignal Value : Subsystem
  _sigControllerOvertempCutback_ : BusSelector  OutputSignals=ISignal Value
  wires:
  sigControllerOvertempCutback/1 -> _sigControllerOvertempCutback_/1  "sigControllerOvertempCutback"
  _sigControllerOvertempCutback_/1 -> ISignal Value/1(ISignal Value)  "<ISignal Value>"

== system DriveSystemControl/Bus Configuration (1) - Out/Simulated ECUs/Virya Controller CAN File 08082024/Telematics/RX/PDUs/TCU03/sigControllerSevereOvertemp ==
  sigControllerSevereOvertemp : Inport
  ISignal Value : Subsystem
  _sigControllerSevereOvertemp_ : BusSelector  OutputSignals=ISignal Value
  wires:
  sigControllerSevereOvertemp/1 -> _sigControllerSevereOvertemp_/1  "sigControllerSevereOvertemp"
  _sigControllerSevereOvertemp_/1 -> ISignal Value/1(ISignal Value)  "<ISignal Value>"

== system DriveSystemControl/Bus Configuration (1) - Out/Simulated ECUs/Virya Controller CAN File 08082024/Telematics/RX/PDUs/TCU03/sigControllerSevereUndertemp ==
  sigControllerSevereUndertemp : Inport
  ISignal Value : Subsystem
  _sigControllerSevereUndertemp_ : BusSelector  OutputSignals=ISignal Value
  wires:
  sigControllerSevereUndertemp/1 -> _sigControllerSevereUndertemp_/1  "sigControllerSevereUndertemp"
  _sigControllerSevereUndertemp_/1 -> ISignal Value/1(ISignal Value)  "<ISignal Value>"
